simulink model "AWES3_CL_wTether_v4_PM"  (R2022a)
settings: Solver=ode3  StartTime=0  StopTime=simInit.TSIM  FixedStep=simInit.dt  RelTol=1e-3
values from neighbouring files (symbols this model uses):
  complex_tether_flag = 1    [run_sim.m]
  Ft_max = 1870    [run_sim.m]
  q = 0    [barrier_optimization.m]
  r = 0    [barrier_optimization.m]
  random_seed = [ 24335       17059       17670        1747]    [run_sim.m]
  safety_controller = false    [run_sim.m]
  turbulence = true    [run_sim.m]
undefined symbols (not defined in the file or in its folder): aeroModel, alpha_max, alpha_min, alpha_options, base_windspeed, constr, DiscIntNeverNeededParam, dx, ENVMT, F, grid_max, grid_min, HDBK, I_table, Light, MIL, mu_max, mu_min, mu_options, P_AP2, params, SampleTime, simInit, T, u0_sim, winchParameter, x0_sim
libraries: simulink x30, aerolibwind2 x14, dspstat3 x2, pid_lib x1, aerolibwindfilters x1, aerolibcommonsys x1, matrix_library x1
(part 4 of 5)

== system AWES3_CL_wTether_v4_PM/FlightController/Retraction/CalculateAttitudeCmds/FlightpathReferenceModels/SecondOrderReferenceModel_Path2 ==
  y_cmd : Inport
  hedge : Inport  Port=2
  Discrete-Time Integrator : DiscreteIntegrator  InitialCondition=30*pi/180  SampleTime=-1  LimitOutput=on  UpperSaturationLimit=y_max  LowerSaturationLimit=y_min  ICPrevOutput=DiscIntNeverNeededParam  ICPrevScaledInput=DiscIntNeverNeededParam
  Discrete-Time Integrator1 : DiscreteIntegrator  SampleTime=-1  LimitOutput=on  UpperSaturationLimit=yd_max  LowerSaturationLimit=yd_min  ICPrevOutput=DiscIntNeverNeededParam  ICPrevScaledInput=DiscIntNeverNeededParam
  Gain1 : Gain  Gain=omega0^2
  Gain2 : Gain  Gain=2*zeta0*omega0
  Saturation : Saturate  UpperLimit=y_max  LowerLimit=y_min
  Saturation1 : Saturate  UpperLimit=y2d_max  LowerLimit=y2d_min
  Sum : Sum  Inputs=|+-
  Sum1 : Sum  Inputs=|+-
  Sum2 : Sum  Inputs=|+-
  y_ref : Outport  VectorParamsAs1DForOutWhenUnconnected=off
  y_ref_dot : Outport  Port=2  VectorParamsAs1DForOutWhenUnconnected=off
  wires:
  hedge/1 -> Sum2/2
  Sum2/1 -> Discrete-Time Integrator/1
  Saturation/1 -> Sum1/1
  Saturation1/1 -> Discrete-Time Integrator1/1
  Sum1/1 -> Gain1/1
  Gain2/1 -> Sum/2
  Sum/1 -> Saturation1/1
  Discrete-Time Integrator1/1 -> Gain2/1, y_ref_dot/1, Sum2/1
  y_cmd/1 -> Saturation/1
  Gain1/1 -> Sum/1
  Discrete-Time Integrator/1 -> Sum1/2, y_ref/1

== system AWES3_CL_wTether_v4_PM/FlightController/Retraction/CalculateAttitudeCmds/FlightpathReferenceModels/SecondOrderReferenceModel_course ==
  y_cmd : Inport
  hedge : Inport  Port=2
  dynamic_pressure : Inport  Port=3
  Constant : Constant  Value=omega0_max
  Constant1 : Constant  Commented=on  Value=omega0_min
  Constant2 : Constant  Commented=on  Value=dynP_min
  Constant3 : Constant  Commented=on  Value=dynP_max
  Discrete-Time Integrator : DiscreteIntegrator  SampleTime=-1  LimitOutput=on  UpperSaturationLimit=y_max  LowerSaturationLimit=y_min  ICPrevOutput=DiscIntNeverNeededParam  ICPrevScaledInput=DiscIntNeverNeededParam
  Discrete-Time Integrator1 : DiscreteIntegrator  SampleTime=-1  LimitOutput=on  UpperSaturationLimit=yd_max  LowerSaturationLimit=yd_min  ICPrevOutput=DiscIntNeverNeededParam  ICPrevScaledInput=DiscIntNeverNeededParam
  Gain2 : Gain  Gain=2*zeta0
  MATLAB Function : MATLAB Function  Commented=on  TreatAsAtomicUnit=on
  Product : Product  Inputs=3
  Product1 : Product
  Saturation : Saturate  UpperLimit=y_max  LowerLimit=y_min
  Saturation1 : Saturate  UpperLimit=y2d_max  LowerLimit=y2d_min
  Saturation2 : Saturate  Commented=on  UpperLimit=dynP_max  LowerLimit=dynP_min
  Sum : Sum  Inputs=|+-
  Sum2 : Sum  Inputs=|+-
  calcualteCourseErrorAndWrap : MATLAB Function  TreatAsAtomicUnit=on
  wrap2pi2 : MATLAB Function  TreatAsAtomicUnit=on
  y_ref : Outport  VectorParamsAs1DForOutWhenUnconnected=off
  y_ref_dot : Outport  Port=2  VectorParamsAs1DForOutWhenUnconnected=off
  wires:
  Product1/1 -> Gain2/1
  Constant2/1 -> MATLAB Function/5(dynP_min)
  Constant1/1 -> MATLAB Function/2(w0_min)
  dynamic_pressure/1 -> Saturation2/1
  Constant/1 -> Product1/2, Product/3, Product/1
  Constant3/1 -> MATLAB Function/4(dynP_max)
  Saturation2/1 -> MATLAB Function/3(dynP)
  Discrete-Time Integrator/1 -> wrap2pi2/1(u)
  Product/1 -> Sum/1
  y_cmd/1 -> Saturation/1
  Discrete-Time Integrator1/1 -> Sum2/1, y_ref_dot/1, Product1/1  "v:_r"
  Sum/1 -> Saturation1/1
  Gain2/1 -> Sum/2
  calcualteCourseErrorAndWrap/1(e_course) -> Product/2
  Saturation1/1 -> Discrete-Time Integrator1/1  "v_dot_r"
  Saturation/1 -> calcualteCourseErrorAndWrap/1(chi_ref)
  Sum2/1 -> Discrete-Time Integrator/1
  hedge/1 -> Sum2/2
  wrap2pi2/1(y) -> calcualteCourseErrorAndWrap/2(chi), y_ref/1

== system AWES3_CL_wTether_v4_PM/FlightController/Retraction/CalculateAttitudeCmds/FlightpathReferenceModels/SecondOrderReferenceModel_mu_a ==
  y_cmd : Inport
  hedge : Inport  Port=2
  reset : Inport  Port=3
  dynamic_pressure : Inport  Port=4
  Constant : Constant  Value=omega0_max
  Constant1 : Constant  Value=omega0_min
  Constant2 : Constant  Value=dynP_min
  Constant3 : Constant  Value=dynP_max
  Discrete-Time Integrator : DiscreteIntegrator  ExternalReset=rising  SampleTime=-1  LimitOutput=on  UpperSaturationLimit=y_max  LowerSaturationLimit=y_min  ICPrevOutput=DiscIntNeverNeededParam  ICPrevScaledInput=DiscIntNeverNeededParam
  Discrete-Time Integrator1 : DiscreteIntegrator  ExternalReset=rising  SampleTime=-1  LimitOutput=on  UpperSaturationLimit=yd_max  LowerSaturationLimit=yd_min  ICPrevOutput=DiscIntNeverNeededParam  ICPrevScaledInput=DiscIntNeverNeededParam
  Gain2 : Gain  Gain=2*zeta0
  MATLAB Function : MATLAB Function  TreatAsAtomicUnit=on
  Product : Product  Inputs=3
  Product1 : Product
  Saturation : Saturate  UpperLimit=y_max  LowerLimit=y_min
  Saturation1 : Saturate  UpperLimit=y2d_max  LowerLimit=y2d_min
  Saturation2 : Saturate  UpperLimit=dynP_max  LowerLimit=dynP_min
  Sum : Sum  Inputs=|+-
  Sum1 : Sum  Inputs=|+-
  Sum2 : Sum  Inputs=|+-
  y_ref : Outport  VectorParamsAs1DForOutWhenUnconnected=off
  y_ref_dot : Outport  Port=2  VectorParamsAs1DForOutWhenUnconnected=off
  wires:
  Saturation2/1 -> MATLAB Function/3(dynP)
  Product1/1 -> Gain2/1
  MATLAB Function/1(w0_int) -> Product1/2, Product/3, Product/1
  Constant3/1 -> MATLAB Function/4(dynP_max)
  Constant2/1 -> MATLAB Function/5(dynP_min)
  Constant/1 -> MATLAB Function/1(w0_max)
  Constant1/1 -> MATLAB Function/2(w0_min)
  dynamic_pressure/1 -> Saturation2/1
  hedge/1 -> Sum2/2
  Sum2/1 -> Discrete-Time Integrator/1
  Saturation/1 -> Sum1/1
  Saturation1/1 -> Discrete-Time Integrator1/1
  Sum1/1 -> Product/2
  Gain2/1 -> Sum/2
  Sum/1 -> Saturation1/1
  Discrete-Time Integrator1/1 -> y_ref_dot/1, Sum2/1, Product1/1
  y_cmd/1 -> Saturation/1
  Product/1 -> Sum/1
  Discrete-Time Integrator/1 -> y_ref/1, Sum1/2
  reset/1 -> Discrete-Time Integrator/2, Discrete-Time Integrator1/2

== system AWES3_CL_wTether_v4_PM/FlightController/Retraction/CalculateAttitudeCmds/FlightpathReferenceModels/SecondOrderReferenceModel_pathangle ==
  y_cmd : Inport
  hedge : Inport  Port=2
  dynamic_pressure : Inport  Port=3
  Constant : Constant  Value=omega0_max
  Constant1 : Constant  Commented=on  Value=omega0_min
  Constant2 : Constant  Commented=on  Value=dynP_min
  Constant3 : Constant  Commented=on  Value=dynP_max
  Discrete-Time Integrator : DiscreteIntegrator  SampleTime=-1  LimitOutput=on  UpperSaturationLimit=y_max  LowerSaturationLimit=y_min  ICPrevOutput=DiscIntNeverNeededParam  ICPrevScaledInput=DiscIntNeverNeededParam
  Discrete-Time Integrator1 : DiscreteIntegrator  SampleTime=-1  LimitOutput=on  UpperSaturationLimit=yd_max  LowerSaturationLimit=yd_min  ICPrevOutput=DiscIntNeverNeededParam  ICPrevScaledInput=DiscIntNeverNeededParam
  Gain2 : Gain  Gain=2*zeta0
  MATLAB Function : MATLAB Function  Commented=on  TreatAsAtomicUnit=on
  Product : Product  Inputs=3
  Product1 : Product
  Saturation : Saturate  UpperLimit=y_max  LowerLimit=y_min
  Saturation1 : Saturate  UpperLimit=y2d_max  LowerLimit=y2d_min
  Saturation2 : Saturate  Commented=on  UpperLimit=dynP_max  LowerLimit=dynP_min
  Sum : Sum  Inputs=|+-
  Sum1 : Sum  Inputs=|+-
  Sum2 : Sum  Inputs=|+-
  y_ref : Outport  VectorParamsAs1DForOutWhenUnconnected=off
  y_ref_dot : Outport  Port=2  VectorParamsAs1DForOutWhenUnconnected=off
  wires:
  Product1/1 -> Gain2/1
  Constant2/1 -> MATLAB Function/5(dynP_min)
  Constant1/1 -> MATLAB Function/2(w0_min)
  dynamic_pressure/1 -> Saturation2/1
  Constant/1 -> Product/3, Product/1, Product1/2
  Constant3/1 -> MATLAB Function/4(dynP_max)
  Saturation2/1 -> MATLAB Function/3(dynP)
  Product/1 -> Sum/1
  y_cmd/1 -> Saturation/1
  Discrete-Time Integrator1/1 -> Sum2/1, y_ref_dot/1, Product1/1  "v:_r"
  Sum/1 -> Saturation1/1
  Gain2/1 -> Sum/2
  Sum1/1 -> Product/2
  Saturation1/1 -> Discrete-Time Integrator1/1  "v_dot_r"
  Saturation/1 -> Sum1/1
  Sum2/1 -> Discrete-Time Integrator/1
  hedge/1 -> Sum2/2
  Discrete-Time Integrator/1 -> y_ref/1, Sum1/2

== system AWES3_CL_wTether_v4_PM/FlightController/Traction/Ft_set_smoothing/force switch1/Subsystem ==
  Ft : Inport
  dFt : Inport  Port=2
  Constant1 : Constant  Value=Ft_max-40
  Gain : Gain  Gain=-1
  Gain1 : Gain  Gain=-1
  Sum : Sum  Inputs=+-|
  Sum1 : Sum  Inputs=+-|
  mu_1 : Outport
  mu_2 : Outport  Port=2
  mu_3 : Outport  Port=3
  mu_4 : Outport  Port=4
  wires:
  Ft/1 -> Sum/2
  Constant1/1 -> Sum/1
  Sum/1 -> Gain/1, Sum1/1, mu_1/1
  dFt/1 -> Sum1/2
  Sum1/1 -> mu_3/1, Gain1/1
  Gain/1 -> mu_2/1
  Gain1/1 -> mu_4/1

== matlab function AWES3_CL_wTether_v4_PM/Aircraft_Winch_Tether/Subsystem/6DoFKinematics1/AircraftEOM2 ==
  data: M_OB output; v_k_W output; v_w_O input; Va input; alpha input; beta input; mu_a input; F_a_A input; chi_a input; gamma_a input; long input; lat input; h_tau input; P_AP2 parameter; pos_O output; pos_W output; v_k_B output; v_a_dot output; chi_a_dot output; gamma_a_dot output; long_dot output; lat_dot output; h_tau_dot output; chi_k output; gamma_k output; eta_EULER output; v_k_O output; ENVMT parameter; course_tau output; pathangle_tau output; beta_k output; EULER_tau output
function [M_OB, v_k_W, pos_O,pos_W, v_k_B, v_a_dot,chi_a_dot,gamma_a_dot,long_dot,lat_dot,h_tau_dot, chi_k, gamma_k,eta_EULER, v_k_O,  course_tau, pathangle_tau, beta_k, EULER_tau] = ...
    fcn(v_w_O,Va, alpha, beta, mu_a, F_a_A , chi_a, gamma_a, long, lat,h_tau, P_AP2, ENVMT)
beta_k= 0;
alpha_k= 0;
chi_k = 0;
gamma_k  = 0;
M_OB = zeros(3); 
eta_EULER = zeros(3,1); 

%cos_a = cos(alpha); 

M_BA = [cos(alpha), 0, -sin(alpha); 
    0, 1, 0; 
 sin(alpha),0, cos(alpha)];

%M_AB = M_BA.';
M_AB = M_BA';

s_lat = sin(lat); 
s_long = sin(long); 
c_lat = cos(lat); 
c_long = cos(long); 

M_tauW = [-s_lat *c_long, -s_lat *s_long, c_lat;
    -s_long, c_long, 0;
    -c_lat*c_long, -c_lat*s_long, -s_lat ];

xi = ENVMT.windDirection_rad;
M_OW = [cos(xi), sin(xi), 0; 
    sin(xi), -cos(xi), 0; 
    0, 0, -1];
M_WO = M_OW; 

cos_ca = cos(chi_a); 
cos_ga = cos(gamma_a); 
sin_ca = sin(chi_a); 
sin_ga = sin(gamma_a); 

M_AbarO = [cos_ca*cos_ga, sin_ca*cos_ga, -sin_ga; 
    -sin_ca, cos_ca, 0; 
    cos_ca*sin_ga, sin_ca*sin_ga, cos_ga];
M_OAbar = M_AbarO';
M_AbarA = [1,0,0; 
            0, cos(mu_a), -sin(mu_a); 
            0, sin(mu_a), cos(mu_a)];
M_AAbar = M_AbarA';

%%

v_a_O = M_OAbar*[Va;0;0]; 
v_a_B = M_BA*[Va;0;0]; 
%v_w_O = M_OW*v_w_W;
v_w_B = M_BA*M_AAbar*M_AbarO*v_w_O;
v_k_B = v_a_B + v_w_B; 
v_k_O = v_a_O + v_w_O; 
v_k_W = M_WO*v_k_O; 
Vk = norm(v_k_B); 
%beta_k = asin(1/Vk * v_k_B(2) );
beta_k = atan2( v_k_B(2), sqrt( v_k_B(1)^2+v_k_B(3)^2 ) );

%alpha_k = atan2( (v_a_B(3)+v_w_B(3)), (v_a_B(1)+v_w_B(1)) );

chi_k = atan2( v_k_O(2), v_k_O(1) ); 
gamma_k = -asin( 1/Vk*v_k_O(3) ); 


Ftot_Abar = M_AbarA*F_a_A; 

x_dot_Abar = 1/P_AP2.mass*diag([1,1/(Va*cos_ga),-1/Va]) * Ftot_Abar; 
% states are: Va, chi_a, gamma_a
v_a_dot = x_dot_Abar(1); 
chi_a_dot = x_dot_Abar(2);
gamma_a_dot = x_dot_Abar(3); 

v_k_tau =M_tauW*v_k_W;

long_dot = v_k_tau(2)/( abs(h_tau)*cos(lat));
lat_dot = v_k_tau(1)/abs(h_tau);
h_tau_dot = -v_k_tau(3);

pos_W= [cos(long)*cos(lat); sin(long)*cos(lat); sin(lat)]*h_tau;
pos_O = M_OW*pos_W; 
M_OB = M_OAbar * M_AbarA * M_AB;
%%

%%
PHI =  atan2( M_OB(3,2), M_OB(3,3) ); 
THETA = -asin( M_OB(3,1) ); 
PSI = atan2( M_OB(2,1), M_OB(1,1) ); 

eta_EULER = [PHI; THETA; PSI];


%% Tangential plane stuff
M_WO=M_OW';  
M_tauB = M_tauW * M_WO * M_OB; 
%phi_tau = atan2( M_tauB(3,2) , M_tauB(3,3) );
phi_tau = atan( M_tauB(3,2)/M_tauB(3,3) );
theta_tau = -asin( M_tauB(3,1) );
psi_tau = atan2( M_tauB(2,1) , M_tauB(1,1) );
EULER_tau = [phi_tau;theta_tau;psi_tau];

vel_k_tau_mDs = M_tauW * M_OW'*M_OB * v_k_B; 
course_tau = atan2( vel_k_tau_mDs(2), vel_k_tau_mDs(1) ); 
pathangle_tau = [course_tau; -asin( vel_k_tau_mDs(3) / norm( vel_k_tau_mDs ) )];

== matlab function AWES3_CL_wTether_v4_PM/Aircraft_Winch_Tether/ForcesAndMoments1/MATLAB Function ==
  data: F_a_A output; airdata input; P_AP2 parameter; F_a_B output; u_trim input
function [F_a_A, F_a_B] = getAeroForcesAndMoments( airdata,  P_AP2, u_trim )
% Rotational Rates
p =0; 
q = 0; %-0.1202; 
r = 0; 

Va = airdata(1); 
beta = airdata(3); 
alpha = airdata(2);

delta_a = 0*u_trim(1); 
delta_e = u_trim(2); % apparently has quite an impact on the Cx coefficient 
delta_r = 0*u_trim(3); 

%% Force coefficients 
% Cx calculation
Cx_0 = P_AP2.Cx_0_0 + P_AP2.Cx_0_alpha * alpha + P_AP2.Cx_0_alpha2 * alpha^2; 
Cx_q = P_AP2.Cx_q_0 + P_AP2.Cx_q_alpha * alpha + P_AP2.Cx_q_alpha2 * alpha^2; 
Cx_deltaE  = P_AP2.Cx_deltaE_0  + P_AP2.Cx_deltaE_alpha * alpha + P_AP2.Cx_deltaE_alpha2 * alpha^2; 
Cx = Cx_0 + Cx_q*P_AP2.c*q/(2*Va) + Cx_deltaE*delta_e; 

% Cy calculation
Cy_beta = P_AP2.Cy_beta_0 + P_AP2.Cy_beta_alpha * alpha + P_AP2.Cy_beta_alpha2 * alpha^2; 
Cy_p = P_AP2.Cy_p_0  + P_AP2.Cy_p_alpha * alpha + P_AP2.Cy_p_alpha2 * alpha^2;  
Cy_r = P_AP2.Cy_r_0  + P_AP2.Cy_r_alpha * alpha + P_AP2.Cy_r_alpha2 * alpha^2;  
Cy_deltaA =P_AP2.Cy_deltaA_0 + P_AP2.Cy_deltaA_alpha * alpha + P_AP2.Cy_deltaA_alpha2 * alpha^2;  
Cy_deltaR =P_AP2.Cy_deltaR_0 + P_AP2.Cy_deltaR_alpha * alpha + P_AP2.Cy_deltaR_alpha2 * alpha^2;  
Cy = Cy_beta*beta + Cy_p*P_AP2.b*p/(2*Va) + Cy_r*P_AP2.b*r/(2*Va) + Cy_deltaA*delta_a + Cy_deltaR*delta_r;


% Cz calculation
Cz_0 = P_AP2.Cz_0_0 + P_AP2.Cz_0_alpha * alpha + P_AP2.Cz_0_alpha2 * alpha.^2; 
Cz_q = P_AP2.Cz_q_0 + P_AP2.Cz_q_alpha * alpha + P_AP2.Cz_q_alpha2 * alpha^2; 
Cz_deltaE  = P_AP2.Cz_deltaE_0 + P_AP2.Cz_deltaE_alpha * alpha + P_AP2.Cz_deltaE_alpha2 * alpha^2; 
Cz = Cz_0 + Cz_q*P_AP2.c*q/(2*Va) + Cz_deltaE*delta_e; 

F_a_B = 0.5*Va^2*P_AP2.S_ref*1.225* [Cx;Cy; Cz];

M_AB = [cos(alpha)*cos(beta), sin(beta), sin(alpha)*cos(beta); 
    -cos(alpha)*sin(beta), cos(beta), -sin(alpha)*sin(beta); 
    -sin(alpha), 0, cos(alpha)];

F_a_A = M_AB * F_a_B;

% Tether drag calculation. Use only the to the tether perpendicular component 
% of the airspeed
% pos_O = transformFromWtoO(windDirection_rad, pos_W);
% Va_B = M_AB'*[Va;0;0];
% Va_O = DCM*Va_B; 
% t_O = pos_O/norm(pos_O); 
% Va_O_parallel = (Va_O'*t_O)*t_O;
% Va_perp_O = Va_O - Va_O_parallel;
% 
% Dt = 1/8*norm(Va_perp_O)^2*1.225*T.d_tether*T.CD_tether*l_tether;
% F_a_tether_A = [-Dt;0;0];

F_a_A = F_a_A; %+ 0*F_a_tether_A; 
%% Moment coefficients

== matlab function AWES3_CL_wTether_v4_PM/Aircraft_Winch_Tether/ForcesAndMoments1/TetherDragApprox ==
  data: Ftd_A output; airdata input; T parameter; pos_W input; M_OB input; Ftd_A2 output; ENVMT parameter
function [Ftd_A, Ftd_A2]  = fcn(airdata,T, pos_W, M_OB,ENVMT)
Ftd_B = zeros(3,1);
windDirection_rad = ENVMT.windDirection_rad; 

long = atan2( pos_W(2), pos_W(1) ); 
lat = asin( pos_W(3)/norm(pos_W) ); 

Va = airdata(1);
alpha = airdata(2);
beta = airdata(3);

%% For test, delete
% long    = -9.568113232685720e-17;
% lat     = 1.396263401595464;
% h_tau   = 250;
% Va      = 31.346599838167194;
% gamma_a = -0.114668330551869;
% chi_a   = -2.210613291576605;
% 
% alpha   = 0.042840397710006;
% mu_a    = 0.083402612962379;
% 
% M_AbarO = [cos(chi_a) .* cos(gamma_a), sin(chi_a) .* cos(gamma_a), -sin(gamma_a); 
%           -sin(chi_a),                 cos(chi_a),                             0; 
%            cos(chi_a) .* sin(gamma_a), sin(chi_a) .* sin(gamma_a), cos(gamma_a)];
% 
% M_OAbar = M_AbarO';
% M_AbarA = [1,0,0;
%            0, cos(mu_a), -sin(mu_a);
%            0, sin(mu_a), cos(mu_a)];
% 
% M_AB = [cos(alpha) .* cos(beta), sin(beta), sin(alpha) .* cos(beta); 
%     -cos(alpha) .* sin(beta), cos(beta), -sin(alpha) .* sin(beta); 
%     -sin(alpha), 0, cos(alpha)];
% 
% M_OB = M_OAbar * M_AbarA * M_AB;


%%


Phi = atan2( M_OB(3,2), M_OB(3,3) );  
Theta = -asin( M_OB(3,1) ); 

M_AB = [cos(alpha)*cos(beta), sin(beta), sin(alpha)*cos(beta);
    -cos(alpha)*sin(beta), cos(beta), -sin(alpha)*sin(beta);
    -sin(alpha), 0, cos(alpha)];

M_BA = M_AB';
v_a_A = [Va;0;0];
v_a_O = M_OB*M_BA*v_a_A; 

gamma_a = -asin( v_a_O(3)/norm(v_a_O) );

mu_a= asin( max( min( (cos(Theta)*sin(Phi))/(cos(gamma_a)*cos(beta)) + tan(gamma_a) * tan(beta), 1),-1) );

Va_W = transformFromOtoW( windDirection_rad, v_a_O);
M_tauW = [-sin(lat)*cos(long), -sin(lat)*sin(long), cos(lat);
    -sin(long), cos(long), 0;
    -cos(lat)*cos(long), -cos(lat)*sin(long), -sin(lat)];
Va_tau= M_tauW*Va_W;

Fd_tau = -1/8*1.225*T.CD_tether*norm(pos_W)*T.d_tether*sqrt( Va_tau(1)^2 + Va_tau(2)^2 ) * [Va_tau(1); Va_tau(2); 0];

Fd_W = M_tauW'*Fd_tau; %transformFromTautoW( long, lat, Fd_tau);
Fd_O = transformFromWtoO(  windDirection_rad, Fd_W);
Ftd_B2 = M_OB'*Fd_O;% transformFromAbar2B(mu_a, alpha, beta, Fd_Abar );

Ftd_A2 = M_AB*Ftd_B2;
%else
%simplified
Fd_Abar = -1/8*1.225*T.CD_tether*norm(pos_W)*T.d_tether*Va * [Va;0;0];
Ftd_B = transformFromAbar2B(mu_a, alpha, beta, Fd_Abar );

Ftd_A = M_AB*Ftd_B;

end

== stateflow chart AWES3_CL_wTether_v4_PM/HighLevelControlSystem/checkRetractionCondition1 ==
  state calcIncrement1
    during: l_tether_predict =l_tether+l_tether-l0;
  state init2
    entry: init_retraction_flag=1;
  state init
    entry: init_retraction_flag=0;
  state calcIncrement
    during: l_tether_predict =l_tether+l_tether-l0;
  state set0length
    entry: l0 = l_tether;
  calcIncrement1 -> (junction 38) : [path_parameter_s >= (3*pi/2+delta_s_1) && path_parameter_s <=3*pi/2+delta_s_2 ]
  init2 -> init : [fm==6]
  (junction 38) -> init2 [order 1] : [l_tether_predict>=l_tether_max]
  set0length -> calcIncrement1 [order 4] : [path_parameter_s >= (pi/2+delta_s_1) && path_parameter_s <= pi/2+delta_s_2]
  (default) -> init
  set0length -> init [order 2] : [fm==6]
  (junction 38) -> set0length [order 2]
  calcIncrement -> (junction 38) : [path_parameter_s >= (pi/2+delta_s_1) && path_parameter_s <= pi/2+delta_s_2]
  set0length -> init [order 3] : [fm==6]
  init -> set0length : [path_parameter_s >= (pi/2+delta_s_1) && path_parameter_s <= pi/2+delta_s_2 &&fm==5]
  set0length -> calcIncrement [order 1] : [path_parameter_s >= (3*pi/2+delta_s_1) && path_parameter_s <=3*pi/2+delta_s_2]
  data: l_tether input; path_parameter_s input; fm input; l0 local; init_retraction_flag output; l_tether_max input; dl local; l_tether_predict local; delta_s_1 parameter; delta_s_2 parameter

== matlab function AWES3_CL_wTether_v4_PM/Aircraft_Winch_Tether/ForcesAndMoments1/allForcesTorques_exceptAero ==
  data: F_A output; P_AP2 parameter; ENVMT parameter; DCM input; F_t_W input; airdata input; pos_W input; F_t_tot input; Ft_flag input; Ftot output


function [F_A,Ftot]      = forces_moments(P_AP2,ENVMT, DCM,F_t_W, airdata, pos_W, F_t_tot, Ft_flag)

Force = zeros(3,1);
beta = airdata(3);
alpha = airdata(2);
% delta_t = 0;
windDirection_rad = ENVMT.windDirection_rad; 
long = atan2( pos_W(2), pos_W(1) ); 
lat = asin( pos_W(3)/norm(pos_W) ); 

if ~Ft_flag % simple tether
    F_t_W = -[cos(long)*cos(lat);
        sin(long)*cos(lat);
        sin(long)]*F_t_tot;
    F_t_W = -pos_W/norm(pos_W)*F_t_tot;
end

Ftot = norm(F_t_W); 

% Complex tether model force in B
f_kite_G_O = transformFromWtoO(windDirection_rad, F_t_W);

%F_tether_vec_B = f_kite_G_B;
%F_prop_B = [delta_t;0;0];
F_prop_B = zeros(3,1);
% last
F_B = DCM'*([0;0;P_AP2.mass*P_AP2.g]+f_kite_G_O) + F_prop_B;

M_AB = [cos(alpha)*cos(beta), sin(beta), sin(alpha)*cos(beta);
    -cos(alpha)*sin(beta), cos(beta), -sin(alpha)*sin(beta);
    -sin(alpha), 0, cos(alpha)];

F_A = M_AB * F_B;




end

== matlab function AWES3_CL_wTether_v4_PM/Aircraft_Winch_Tether/WindfieldModel/Subsystem1/MATLAB Function1 ==
  data: u input; y output; windDir input
function y = fcn(u, windDir)

%y = transformFromOtoW(windDir,u);

y = zeros(3,1);
M_WO = [cos(windDir), sin(windDir), 0;
        sin(windDir), -cos(windDir), 0;
        0, 0, -1];

y = M_WO*u;

% y(1) = -y(1); 
 %y(3) = -y(3);

== matlab function AWES3_CL_wTether_v4_PM/Aircraft_Winch_Tether/WindfieldModel/Subsystem1/MATLAB Function2 ==
  data: u input; y output; windDir input
function y = fcn(u, windDir)

%y = transformFromOtoW(windDir,u);

y = zeros(3,1);
M_WO = [cos(windDir), sin(windDir), 0;
        sin(windDir), -cos(windDir), 0;
        0, 0, -1];

y = M_WO*u;

% y(1) = -y(1); 
 %y(3) = -y(3);

== matlab function AWES3_CL_wTether_v4_PM/Power/MATLAB Function ==
  data: flag input; m_old input; p_sum input; cnt input; u input; flag output; flightMode input; e_old input; cnt_max_mat input; cycles_cnt input; m_new output; p_sum output; cnt output; e_new output; cnt_max_mat output; cycles_cnt output
% Copyright 2021 Delft University of Technology
%
% Licensed under the Apache License, Version 2.0 (the "License");
% you may not use this file except in compliance with the License.
% You may obtain a copy of the License at
%
%      http://www.apache.org/licenses/LICENSE-2.0
%
% Unless required by applicable law or agreed to in writing, software
% distributed under the License is distributed on an "AS IS" BASIS,
% WITHOUT WARRANTIES OR CONDITIONS OF ANY KIND, either express or implied.
% See the License for the specific language governing permissions and
% limitations under the License.

function [flag, m_new, p_sum, cnt, e_new, cnt_max_mat,cycles_cnt] = fcn(flag, m_old, p_sum, cnt, u, flightMode, e_old,cnt_max_mat,cycles_cnt)

p_sum = p_sum + u;
cnt = cnt + 1;

if flightMode == 5 && flag
    % entering Traction
    cnt_max_mat = cnt; 
    m_new = p_sum/cnt;
    cnt  = 0;
    cycles_cnt = cycles_cnt + 1;
    p_sum = 0;
    flag = 0;
    e_new = abs( m_new - m_old );
elseif flightMode == 6 || flightMode == 7
    % Retraction
    flag = 1;
    m_new = m_old;
    e_new = e_old;
else
    % first Traction
    flag = 0;
    m_new = m_old;
    e_new = e_old;
end

== matlab function AWES3_CL_wTether_v4_PM/FlightController/Traction/Ft_set_smoothing/force switch1/MATLAB Function ==
  data: mu1 input; sigma output; mu2 input; mu3 input; mu4 input; sigma input
function sigma = switching(mu1, mu2, mu3, mu4, sigma)
% sigma = 0: NDI
% sigma = 1: safety
h = 0.10;

if sigma == 0
    if mu1*(1+h) <= min(mu2, mu4) || ...
        mu3*(1+h) <= min(mu2, mu4)
        sigma = 1;
    end
else
    if mu2*(1+h) <= min(mu1, mu3) || ...
        mu4*(1+h) <= min(mu1, mu3)
        sigma = 0;
    end
end

== matlab function AWES3_CL_wTether_v4_PM/FlightController/Traction/Subsystem3/Safety control ==
  data: value output; s input; mu_a output; sigma input; h_tau input; Va input; chi_a input; gamma_a input; tether_diff input; alpha_a output; alpha_options parameter; mu_options parameter; alpha_max parameter; grid_min parameter; grid_max parameter; dx parameter; mu_max parameter; I_table parameter; alpha_min parameter; mu_min parameter
function [value, mu_a, alpha_a] = safetyControl(s, sigma, h_tau, Va, chi_a, gamma_a, tether_diff, alpha_options, mu_options, alpha_max, grid_min, grid_max, dx, mu_max, I_table, alpha_min, mu_min)

    x       = [s, sigma, h_tau, Va, chi_a, gamma_a, tether_diff];
    boundary_min = grid_min' > x;
    boundary_max = grid_max' < x;
    if any(boundary_min) || any(boundary_max)
        value   = false;
        alpha_a = 0;
        mu_a    = 0;
        return
    end
    
    value = true;

    I = eval_u(grid_min, grid_max, dx, I_table, x, 'nearest');
    [I1,I2] = ind2sub([alpha_options, mu_options], I);
    
    alpha_a = alpha_min + (I1-1)/(alpha_options-1) * (alpha_max - alpha_min);
    mu_a    = mu_min    + (I2-1)/(mu_options   -1) * (mu_max    - mu_min);
end    
function v = eval_u(grid_min, grid_max, dx, datas, xs, interp_method)
% Only supporting Single grid, single value function, multiple states
    if nargin < 4
      interp_method = 'linear';
    end
    v = eval_u_single(grid_min, grid_max, dx, datas, xs, interp_method);
end

function v = eval_u_single(grid_min, grid_max, dx, data, x, interp_method)
% v = eval_u_single(g, data, x)
%   Computes the interpolated value of a value function data at state x
%
% Inputs:
%   g       - grid
%   data    - implicit function describing the set
%   x       - points to check; each row is a point
%
% OUTPUT
%   v:  value at points x


%% Dealing with periodicity
% Not implementing now, but should be handled

%% Interpolate
% Input checking
%x = checkInterpInput(g, x);

% Hardcoded for 7 states for now
VS_1 = (grid_min(1) : dx(1) : grid_max(1))';
VS_2 = (grid_min(2) : dx(2) : grid_max(2))';
VS_3 = (grid_min(3) : dx(3) : grid_max(3))';
VS_4 = (grid_min(4) : dx(4) : grid_max(4))';
VS_5 = (grid_min(5) : dx(5) : grid_max(5))';
VS_6 = (grid_min(6) : dx(6) : grid_max(6))';
VS_7 = (grid_min(7) : dx(7) : grid_max(7))';

v = interpn(VS_1, VS_2, VS_3, VS_4, VS_5, VS_6, VS_7, data, ...
            x(1), x(2), x(3), x(4), x(5), x(6), x(7), interp_method);

end

== matlab function AWES3_CL_wTether_v4_PM/Aircraft_Winch_Tether/WindfieldModel/MATLAB Function1 ==
  data: wind_direction_rad input; vec_O output; vec_W input
function vec_O = fcn(wind_direction_rad, vec_W)


M_WO = [cos(wind_direction_rad), sin(wind_direction_rad), 0;
        sin(wind_direction_rad), -cos(wind_direction_rad), 0;
        0, 0, -1];

vec_O = M_WO' * vec_W;

== matlab function AWES3_CL_wTether_v4_PM/Aircraft_Winch_Tether/Subsystem1/MATLAB Function ==
  data: s_dot output; sigma_dot output; F_t_W input; s input; sigma input; long_alt input; lat_alt input; h_tau input; va input; chi_a input; gamma_a input; tether_diff input; alpha input; mu_a input; tether_diff_dot input; v_w_O input; PHI_BOOTH input; long_dot output; lat_dot output; h_tau_dot output; va_dot output; chi_a_dot output; gamma_a_dot output; tether_diff_dot output; T parameter; ENVMT parameter; P_AP2 parameter; base_windspeed parameter; params parameter; F_rest_Abar output
function [s_dot, sigma_dot, long_dot, lat_dot, h_tau_dot, va_dot, chi_a_dot, gamma_a_dot, tether_diff_dot, F_rest_Abar] = ...
    safety_critical_dynamics(F_t_W, s, sigma, long_alt, lat_alt, h_tau, va, chi_a, gamma_a, tether_diff, alpha, mu_a, tether_diff_dot, v_w_O, PHI_BOOTH, T, ENVMT, P_AP2, base_windspeed, params)

% long     = x(1);
% lat      = x(2);
% h_tau    = x(3);
% va       = x(4);
% chi_a    = x(5);
% gamma_a  = x(6);
% tether_diff  = x(7);
% 
% alpha    = u(1);
% mu_a     = u(2);
% l_s_dot  = u(3);
direction = params.direction;
[long, lat, t_tau, t_rot_tau] = getLongLat(s, sigma, h_tau, PHI_BOOTH, params);
% 
% if retraction_flag
%     long = long_alt;
%     lat = lat_alt;
% end
    long = long_alt;
    lat = lat_alt;

beta     = 0;
% Rotational Rates
p = 0; 
q = 0;
r = 0; 

% Hardcoded for now
delta_a = 0; 
delta_e = -0.092174717977942;
delta_r = 0; 

xi      = ENVMT.windDirection_rad;

%% Define rotation matrix
M_AbarA = [1,0,0; 
           0, cos(mu_a), -sin(mu_a); 
           0, sin(mu_a), cos(mu_a)];

M_AB = [cos(alpha) .* cos(beta), sin(beta), sin(alpha) .* cos(beta); 
    -cos(alpha) .* sin(beta), cos(beta), -sin(alpha) .* sin(beta); 
    -sin(alpha), 0, cos(alpha)];

%% Force coefficients 
% Cx calculation
Cx_0 = P_AP2.Cx_0_0 + P_AP2.Cx_0_alpha * alpha + P_AP2.Cx_0_alpha2 * alpha.^2; 
Cx_q = P_AP2.Cx_q_0 + P_AP2.Cx_q_alpha * alpha + P_AP2.Cx_q_alpha2 * alpha.^2; 
Cx_deltaE  = P_AP2.Cx_deltaE_0  + P_AP2.Cx_deltaE_alpha * alpha + P_AP2.Cx_deltaE_alpha2 * alpha.^2; 
Cx = Cx_0 + Cx_q*P_AP2.c*q./(2*va) + Cx_deltaE*delta_e; 

% Cy calculation
Cy_beta = P_AP2.Cy_beta_0 + P_AP2.Cy_beta_alpha * alpha + P_AP2.Cy_beta_alpha2 * alpha.^2; 
Cy_p = P_AP2.Cy_p_0  + P_AP2.Cy_p_alpha * alpha + P_AP2.Cy_p_alpha2 * alpha.^2;  
Cy_r = P_AP2.Cy_r_0  + P_AP2.Cy_r_alpha * alpha + P_AP2.Cy_r_alpha2 * alpha.^2;  
Cy_deltaA = P_AP2.Cy_deltaA_0 + P_AP2.Cy_deltaA_alpha * alpha + P_AP2.Cy_deltaA_alpha2 * alpha.^2;  
Cy_deltaR = P_AP2.Cy_deltaR_0 + P_AP2.Cy_deltaR_alpha * alpha + P_AP2.Cy_deltaR_alpha2 * alpha.^2;  
Cy = Cy_beta*beta + Cy_p*P_AP2.b*p./(2*va) + Cy_r*P_AP2.b*r./(2*va) + Cy_deltaA*delta_a + Cy_deltaR*delta_r;

% Cz calculation
Cz_0 = P_AP2.Cz_0_0 + P_AP2.Cz_0_alpha * alpha + P_AP2.Cz_0_alpha2 * alpha.^2; 
Cz_q = P_AP2.Cz_q_0 + P_AP2.Cz_q_alpha * alpha + P_AP2.Cz_q_alpha2 * alpha.^2; 
Cz_deltaE  = P_AP2.Cz_deltaE_0 + P_AP2.Cz_deltaE_alpha * alpha + P_AP2.Cz_deltaE_alpha2 * alpha.^2; 
Cz = Cz_0 + Cz_q*P_AP2.c*q./(2*va) + Cz_deltaE*delta_e; 

%% Translation Dynamics 
M_tauW = [-sin(lat) .* cos(long), -sin(lat) .* sin(long), cos(lat);
          -sin(long)            , cos(long)             , 0;
          -cos(lat) .* cos(long), -cos(lat) .* sin(long), -sin(lat) ];

M_AbarO = [cos(chi_a) .* cos(gamma_a), sin(chi_a) .* cos(gamma_a), -sin(gamma_a); 
          -sin(chi_a),                 cos(chi_a),                             0; 
           cos(chi_a) .* sin(gamma_a), sin(chi_a) .* sin(gamma_a), cos(gamma_a)];
M_OAbar = M_AbarO';

M_OW = [cos(xi),  sin(xi),  0; 
        sin(xi), -cos(xi),  0; 
        0,              0, -1];
M_WO = M_OW; 

v_a_O = M_OAbar * [va;0;0];
v_k_O = v_a_O + v_w_O; 
v_k_W = M_WO * v_k_O; 

v_k_tau = M_tauW * v_k_W;


s_dot     = 2*pi/945 * t_tau'*v_k_tau./ (direction*norm(t_tau));
sigma_dot = t_rot_tau'*v_k_tau./ (norm(t_tau));

long_dot = (v_k_tau(2))./( abs(h_tau).*cos(lat));
lat_dot = (v_k_tau(1))./abs(h_tau);
h_tau_dot = -(v_k_tau(3));

[pos_W_x,pos_W_y,pos_W_z] = sph2cart(long, lat, h_tau);
pos_W = [pos_W_x; pos_W_y; pos_W_z];
%% Calculate Aerodynamic Forces and Moments
F_a_B = 0.5 * P_AP2.S_ref * 1.225*(va).^2 * [Cx;Cy; Cz];
F_a_A = M_AB * F_a_B;

%% All Forces except Aero
% x_W = [long; lat; h_tau; long_dot; lat_dot; h_tau_dot; tether_diff];
% [f_kite_G_approx , final_seg_diff_dot] = tether_forces(x_W, P_AP2, ENVMT, T, base_windspeed);
%tether_diff_dot = final_seg_diff_dot - l_s_dot;
% F_t_W_approx = -1 * f_kite_G_approx;

%tether_diff_dot = 0;
f_kite_G_O= M_OW * F_t_W;
F_rest_Abar = M_AbarO * ([0;0;P_AP2.mass * ENVMT.g] + f_kite_G_O);

%% Combine all forces
Ftot_Abar = M_AbarA * F_a_A + F_rest_Abar;

va_dot = 1/P_AP2.mass * Ftot_Abar(1);
chi_a_dot  = 1/P_AP2.mass * 1/(va .* cos(gamma_a)) .* Ftot_Abar(2);
gamma_a_dot = 1/P_AP2.mass * -1/(va) .* Ftot_Abar(3);

== matlab function AWES3_CL_wTether_v4_PM/Aircraft_Winch_Tether/Bus Selector/MATLAB Function1 ==
  data: M_OB output; long input; lat input; h_tau input; Va input; chi_a input; gamma_a input; v_k_W output; pos_O output; pos_W output; v_k_B output; Va output; chi_a output; gamma_a output; long output; lat output; h_tau output; chi_k output; gamma_k output; eta_EULER output; v_k_O output; pathangle_tau output; EULER_tau output; alpha_a input; mu_a input; v_w_O input; alpha_a output; ENVMT parameter
function [M_OB, v_k_W, pos_O,pos_W, v_k_B, Va,chi_a,gamma_a,long,lat,h_tau, chi_k, gamma_k,eta_EULER, v_k_O,  pathangle_tau, EULER_tau, alpha_a] = ...
    AricraftBus( long, lat,h_tau, Va, chi_a, gamma_a, alpha_a, mu_a, v_w_O, ENVMT)


M_BA = [cos(alpha_a), 0, -sin(alpha_a); ...
            0, 1, 0; ...
         sin(alpha_a),0, cos(alpha_a)];
M_AB = M_BA';

s_lat = sin(lat); 
s_long = sin(long); 
c_lat = cos(lat); 
c_long = cos(long); 

M_tauW = [-s_lat *c_long, -s_lat *s_long, c_lat;...
    -s_long, c_long, 0;...
    -c_lat*c_long, -c_lat*s_long, -s_lat ];

xi = ENVMT.windDirection_rad;
M_OW = [cos(xi), sin(xi), 0; 
    sin(xi), -cos(xi), 0; 
    0, 0, -1];
M_WO = M_OW; 

cos_ca = cos(chi_a); 
cos_ga = cos(gamma_a); 
sin_ca = sin(chi_a); 
sin_ga = sin(gamma_a); 

M_AbarO = [cos_ca*cos_ga, sin_ca*cos_ga, -sin_ga;  ...
    -sin_ca, cos_ca, 0; ...
    cos_ca*sin_ga, sin_ca*sin_ga, cos_ga];
M_OAbar = M_AbarO';
M_AbarA = [1,0,0; 
            0, cos(mu_a), -sin(mu_a); 
            0, sin(mu_a), cos(mu_a)];
M_AAbar = M_AbarA';

%%

v_a_O = M_OAbar*[Va;0;0]; 
v_a_B = M_BA*[Va;0;0]; 
%v_w_O = M_OW*v_w_W;
v_w_B = M_BA*M_AAbar*M_AbarO*v_w_O;
v_k_B = v_a_B + v_w_B; 
v_k_O = v_a_O + v_w_O; 
v_k_W = M_WO*v_k_O; 
Vk = norm(v_k_B); 

chi_k = atan2( v_k_O(2), v_k_O(1) );
if abs(1/Vk*v_k_O(3)) > 1
    gamma_k = -asin( max(min(1/Vk*v_k_O(3), 1), -1) );
else
    gamma_k = -asin( 1/Vk*v_k_O(3) ); 
end

pos_W= [cos(long)*cos(lat); sin(long)*cos(lat); sin(lat)]*h_tau;
pos_O = M_OW*pos_W; 
M_OB = M_OAbar * M_AbarA * M_AB;

PHI =  atan2( M_OB(3,2), M_OB(3,3) ); 
THETA = -asin( M_OB(3,1) ); 
PSI = atan2( M_OB(2,1), M_OB(1,1) ); 

eta_EULER = [PHI; THETA; PSI];

%% Tangential plane stuff
M_WO=M_OW';  
M_tauB = M_tauW * M_WO * M_OB; 
%phi_tau = atan2( M_tauB(3,2) , M_tauB(3,3) );
phi_tau = atan( M_tauB(3,2)/M_tauB(3,3) );
theta_tau = -asin( M_tauB(3,1) );
psi_tau = atan2( M_tauB(2,1) , M_tauB(1,1) );
EULER_tau = [phi_tau;theta_tau;psi_tau];

vel_k_tau_mDs = M_tauW * M_OW'*M_OB * v_k_B; 
course_tau = atan2( vel_k_tau_mDs(2), vel_k_tau_mDs(1) ); 
pathangle_tau = [course_tau; -asin( vel_k_tau_mDs(3) / norm( vel_k_tau_mDs ) )]; 
end

== matlab function AWES3_CL_wTether_v4_PM/Aircraft_Winch_Tether/WindfieldModel/Subsystem1/MATLAB Function ==
  data: u input; y output; windDir input
function y = fcn(u, windDir)

%y = transformFromOtoW(windDir,u);

y = zeros(3,1);
M_WO = [cos(windDir), sin(windDir), 0;
        sin(windDir), -cos(windDir), 0;
        0, 0, -1];

y = M_WO*u;

% y(1) = -y(1); 
 %y(3) = -y(3);

== matlab function AWES3_CL_wTether_v4_PM/Aircraft_Winch_Tether/ParticleTetherModel/Tethermodel ==
  data: x_dot input; x_dotdot_TetherG2K output; x input; v_ro_set input; l_s input; pos_G_W input; vel_k_G_W input; landedFlag input; l_s_dot output; ground_tether_force output; ENVMT parameter; T parameter; f_kite_G output; vel_W_W_mat input; P_AP2 parameter
function [x_dotdot_TetherG2K,l_s_dot, ground_tether_force,f_kite_G]    = pure_tether_model_function(x_dot, x,...
    v_ro_set,l_s, pos_G_W,vel_k_G_W, landedFlag,ENVMT, T, vel_W_W_mat,P_AP2)
%% Readme
% Equations are adapted from Fechner et al, Dynamic Model of a Pumping Kite
% Power System, Renewable Energy, 2015.
% Implementation: Sebastian Rapp, Wind Energy Institute, Faculty of
% Aerospace Engineering, TU Delft
% Mail: s.rapp@tudelft.nl
% Last change: 19.01.2018
%
% General description:
% This functions calculates the accelerations of the tether particle
% segment based on the acting forces at each particle.
%
% Inputs:
% x_dot: Tether particle velocities (world frame i.e. inertial frame)
% x: Tether particle position (world frame)
% v_w: wind vector (world frame)
% d_tether: tether diameter
% CD_tether: tether drag coefficient
% v_ro_set: reelout speed of the tether
% l_s: tether segment length
% c0: intial spring constant of a tether segment
% d0: initial damping constant of a tether segment
% rho_t: tether mass density (i.e. mass per m)
% g_vec: gravity vector
% rho_air: air density
% x_kite_A,C,D: position bridle attachment points
% xdot_kite_A,C,D: velocities of bridle attachment points
% ls_AKcu,CKcu,DKcu: bridle lengths
% m_kcu: kcu weight
%
% Outputs:
% x_dotdot_TetherG2K: accelertions of the tether particles
% l_s_dot: tether length increases with this speed
% ground_tether_force: tether force as measured at the ground



c0 = T.c0;
d0 = T.d0;
rho_t = P_AP2.rho_tether;% T.rho_t; 
d_tether = P_AP2.d_tether;%  T.d_tether;
CD_tether = P_AP2.Cd_tether;% T.CD_tether;

n_t_p = 5; % amount of particles
l_s_dot = v_ro_set/(n_t_p+1); % Particle speeds

% Adapt stiffness and damping with respect to current segment length
c = c0/max(l_s,60);
d = d0/max(l_s,60);

c = c0/60; 
d = d0/60;

% Mass of tether segments with  respect to current segment length
m = l_s * rho_t;
m_vec = m * ones(n_t_p,1);
%m_vec(n_t_p) = (l_s/2 * rho_t);

p_vec = x;
v_vec = x_dot;
p_norm = zeros(n_t_p,1);

% Vector with distances between particles
p_d = p_vec - [0;0;0; p_vec(1:3*n_t_p-3)];

% Vector with velocity differences
v_d = v_vec - [0;0;0; v_vec(1:3*n_t_p-3)];
%v_d = v_vec - [p_d(1:3)*l_s_dot; v_vec(1:3*n_t_p-3)];

% calculate absolute distances between points
for iter = 1 : n_t_p
    p_norm(iter) = norm( p_d( (iter-1)* 3 + 1 : (iter-1) * 3 + 3 ) );
end

% Gravity vector in W frame
g_vec = [0;0;ENVMT.g];

%%------------------------------- Set up equations of motion-------------------------------
% Initialize matrices
fsd_tot_mat = zeros(3,n_t_p);
x_dotdot = zeros(3,n_t_p);
D_s_mat = zeros(3,n_t_p);

%% Set up equations of motions of ground to kite tether

% Boundary tether force from kite to particle below kite (in the 4p kite model the kcu is connected to the
% points A, C and D

f_kite_G = calcSpringDamperForce( c0,norm( pos_G_W - p_vec(3*(n_t_p) -2 : 3*(n_t_p) ) ), l_s, d0,...
    pos_G_W - p_vec(3*(n_t_p) -2 : 3*(n_t_p) ) ,...
    vel_k_G_W - v_vec( 3*(n_t_p) -2 : 3*(n_t_p)  ) );

 
v_a_p_save = zeros(3, n_t_p);

% Loop through all particles
for idx = 1 : n_t_p
    %v_w_vec = [v_w( idx,: );0;0]+turbulence;
    v_w_vec = vel_W_W_mat(:,idx);
    % Calculate Spring-Damper forces
    fsd_tot_mat(:,idx) = calcSpringDamperForce( c, p_norm(idx), l_s, d, p_d( (idx-1)*3+1:(idx-1)*3+3 ), v_d( (idx-1)*3+1:(idx-1)*3+3) );
    if idx < n_t_p
        fsd_tot_mat(:,idx+1) = calcSpringDamperForce( c, p_norm(idx+1), l_s, d, p_d( idx*3+1:idx*3+3 ), v_d( idx*3+1:idx*3+3) );
    end
    
    % Calculate apparent wind speed of tether particles
    if idx == 1 % Segment that is connected to the ground
        v_a_p = v_w_vec - 0.5*x_dot(1:3) ;
    elseif idx == n_t_p
        v_a_p = v_w_vec - 0.5*( x_dot((idx-2)*3+1:(idx-2)*3+3) + x_dot( (idx-1)*3+1:(idx-1)*3+3) ); % take mean value of adjacent particle vel. for segment velocity
    else
        v_a_p = v_w_vec - 0.5*( x_dot((idx-2)*3+1:(idx-2)*3+3) + x_dot( (idx-1)*3+1:(idx-1)*3+3) ); % take mean value of adjacent particle vel. for segment velocity
    end
    v_a_p_save(1:3, idx) = v_a_p;
    
    % Calculate segment drag
    D_s_mat(:,idx) = 1*calcSegmentDrag(p_d((idx-1)*3+1:(idx-1)*3+3) , v_a_p, ENVMT.rhos, CD_tether, d_tether); % segment drag
    if idx < n_t_p
        % Equations of motion for the groud tether particles Newton x_dotdot = 1/m * (-f + u -mg )
        if idx+1 == n_t_p
            x_dotdot(:,idx) = 1/m_vec(idx) * ( -fsd_tot_mat(:,idx) + 1*fsd_tot_mat(:,idx+1) - m_vec(idx)*g_vec  + D_s_mat(:,idx) );  % Particle dynamics
        else
            if idx == 1
                x_dotdot(:,idx) = 1/m_vec(idx) * ( -fsd_tot_mat(:,1) + fsd_tot_mat(:,2) - m_vec(1)*g_vec  + D_s_mat(:,1) );  % Particle dynamics
            else
                x_dotdot(:,idx) = 1/m_vec(idx) * ( -fsd_tot_mat(:,idx) + 1*fsd_tot_mat(:,idx+1) - m_vec(idx)*g_vec  + D_s_mat(:,idx) );  % Particle dynamics
            end
        end
    else
        % Flexible tether: last particle of the tether is connected to the
        % aircraft CG.
        x_dotdot(:,idx) = 1/m_vec(idx) * ( -1*fsd_tot_mat(:,idx) + f_kite_G - m_vec(idx)*g_vec  + D_s_mat(:,idx) );  % Particle dynamics
    end
    
    ground_tether_force =  fsd_tot_mat(:,1);
    
end

x_dotdot_TetherG2K = reshape(x_dotdot, [3*n_t_p,1]);
if landedFlag
    x_dotdot_TetherG2K = 0 * x_dotdot_TetherG2K;
end


end

== matlab function AWES3_CL_wTether_v4_PM/Aircraft_Winch_Tether/WindfieldModel/MATLAB Function ==
  data: wind_direction_rad input; vec_W output; vec_O input
function vec_W = fcn(wind_direction_rad, vec_O)

vec_W = transformFromOtoW(wind_direction_rad, vec_O);

== matlab function AWES3_CL_wTether_v4_PM/Aircraft_Winch_Tether/WindfieldModel/ShearWind/MATLAB Function ==
  data: v_w_u input; v_w_p_mat output
function v_w_p_mat = fcn(v_w_u)

v_w_p_mat = zeros( 3, length( v_w_u) );
v_w_p_mat(1,:) = v_w_u';

== stateflow chart AWES3_CL_wTether_v4_PM/HighLevelControlSystem/Chart ==
  state AvoidanceFtRup
    entry: mode = 5;
    entry: pathRotFlag = 1;
    during: Ft_set = Ft_set_avoidance;
    during: Pacc = (Pacc+Pin/cnt)*cnt/(cnt+1);
    during: vr_acc = (vr_acc+vr_in);
    during: vr_mean = vr_acc/cnt;
    during: vr_mean_out = vr_mean;
    during: cnt = cnt + 1;
    entry: Ft_set_init = Ft_set_avoidance;
  state StopSim2
    entry:stopSimFlag=1;
  state initTRACTION
    entry: mode = 5;
    entry: cnt = 1;
    entry: Pacc = 0;
    entry: pathRotFlag = 0;
    entry: cycleCounter = 0;
    entry: trac_count = 0;
    during: Ft_set = Ft_set_traction;
    during: Pacc = (Pacc+Pin/cnt)*cnt/(cnt+1);
    during: cnt = cnt + 1;
    entry: Ft_set_init = 1000;
  state TRACTION
    entry: mode = 5;
    entry: pathRotFlag = 1;
    during: Ft_set = Ft_set_traction;
    during: Pacc = (Pacc+Pin/cnt)*cnt/(cnt+1);
    during: vr_acc = (vr_acc+vr_in);
    during: vr_mean = vr_acc/cnt;
    during: vr_mean_out = vr_mean;
    during: cnt = cnt + 1;
  state RETRACTION
    entry: mode = 6;
    during: Ft_set = Ft_set_retraction;
    during: Pacc = (Pacc+Pin/cnt)*cnt/(cnt+1);
    during: cnt = cnt + 1;
    entry: Ft_set_init = Ft_set_retraction;
  state Trans
    entry: trac_count = trac_count + 1;
    entry: mode = 4;
    entry: Ft_set = Ft_set_retraction;
    during: Pacc = (Pacc+Pin/cnt)*cnt/(cnt+1);
    during: cnt = cnt + 1;
  state ApproachTraction
    entry: mode = 7;
    entry: Ft_set = Ft_set_traction;
    entry: Pacc = (Pacc+Pin/cnt)*cnt/(cnt+1);
    entry: cnt = cnt + 1;
    entry: e=abs(Pacc-P_mean_old);
    entry: e_out = e;
    during: Ft_set = Ft_set_traction;
    during: Pacc = (Pacc+Pin/cnt)*cnt/(cnt+1);
    during: cnt = cnt + 1;
    during: e=abs(Pacc-P_mean_old);
    exit: P_mean_old = Pacc;
    exit: cycleCounter = cycleCounter + 1;
    exit: cycleCounter_log = cycleCounter;
  state initTRACTION_4
    entry: mode = 5;
    entry: cnt = 1;
    entry: Pacc = 0;
    entry: pathRotFlag = 0;
    during: Ft_set = Ft_set_traction;
    during: Pacc = (Pacc+Pin/cnt)*cnt/(cnt+1);
    during: cnt = cnt + 1;
  state StopSim1
    entry:stopSimFlag=1;
  TRACTION -> AvoidanceFtRup [order 2] : [avoid_flag==1]
  AvoidanceFtRup -> TRACTION : [avoid_flag==0]
  Trans -> StopSim2 [order 2] : [trac_count>=trac_count_max]
  initTRACTION -> TRACTION : [mod(s,pi)<0.1]
  (default) -> initTRACTION
  Trans -> RETRACTION [order 1] : [Ft<Ft_set_traction*0.8]
  TRACTION -> Trans [order 1] : [initRetractionFlag==1]
  initTRACTION_4 -> TRACTION [order 1] : [mod(s,pi)<0.01]
  RETRACTION -> ApproachTraction : [approachFlag==1]
  ApproachTraction -> initTRACTION_4 : [initTractionFlag==1&&l_t<l_t_min_max]
  initTRACTION_4 -> StopSim1 [order 2] : [cycleCounter>=cycleCounterMax]
  data: initRetractionFlag input; initTractionFlag input; Ft_set output; mode output; Ft_set_traction parameter; Ft_set_retraction parameter; l_t input; l_t_min_max parameter; Ft input; cnt local =1; P_mean_old local =constr.F_t_max*constr.winchParameter.v_max*0.001; Pacc local =0; Pin input; s input; pathRotFlag output; cycleCounterMin parameter; e_conv parameter; stopSimFlag output; cycleCounter local; e local; approachFlag input; cycleCounter_log output; cycleCounterMax parameter; e_out output; vr_in input; Ft_set_traction_low parameter; vr_mean_min parameter; path_rot_complete_flag input; vr_mean local =0; vr_acc local =0; vr_mean_out output; Ft_set_avoidance parameter; avoid_flag input; Ft_set_init output; trac_count local; trac_count_max parameter

== stateflow chart AWES3_CL_wTether_v4_PM/HighLevelControlSystem/checkRetractionCondition ==
  state calcIncrement1
    during: l_tether_predict =l_tether+l_tether-l0;
    during: initiate_trans_retraction_flag = l_tether_predict>=l_tether_max;
  state set0length
    entry: l0 = l_tether;
  state init2
    entry: init_retraction_flag=1;
  state init
    entry: init_retraction_flag=0;
  state calcIncrement
    during: l_tether_predict =l_tether +l_tether-l0;
    during: initiate_trans_retraction_flag = l_tether_predict>=l_tether_max;
  set0length -> calcIncrement1 [order 3] : [path_parameter_s >= (pi/2+delta_s_1) && path_parameter_s <= pi/2+delta_s_2]
  calcIncrement1 -> (junction 38) : [path_parameter_s >= (3*pi/2+delta_s_1) && path_parameter_s <=3*pi/2+delta_s_2 ]
  (junction 38) -> set0length [order 2]
  (junction 38) -> init2 [order 1] : [l_tether_predict>=l_tether_max]
  set0length -> init [order 2] : [fm==6]
  calcIncrement -> (junction 38) : [path_parameter_s >= (pi/2+delta_s_1) && path_parameter_s <= pi/2+delta_s_2]
  (default) -> init
  init2 -> init : [fm==6]
  init -> set0length : [path_parameter_s >= (pi/2+delta_s_1) && path_parameter_s <= pi/2+delta_s_2 &&fm==5]
  set0length -> calcIncrement [order 1] : [path_parameter_s >= (3*pi/2+delta_s_1) && path_parameter_s <=3*pi/2+delta_s_2]
  data: l_tether input; path_parameter_s input; fm input; l0 local; init_retraction_flag output; l_tether_max input; dl local; l_tether_predict local; delta_s_1 parameter; delta_s_2 parameter; initiate_trans_retraction_flag output

== stateflow chart AWES3_CL_wTether_v4_PM/HighLevelControlSystem/Init_Solutions ==
  state SimInit1
    entry: s_init = 3/2*pi;
  state SimInit
    entry: s_init = 2*pi;
  state SimInit2
    entry: s_init = pi/2;
  SimInit1 -> (junction 8) : [mode==6]
  (junction 8) -> SimInit1 [order 1] : [long<=0]
  SimInit -> (junction 8) : [mode==6]
  (default) -> SimInit
  (junction 8) -> SimInit2 [order 2] : [long>0]
  SimInit2 -> (junction 8) : [mode==6]
  data: mode input; long input; s_init output

== matlab function AWES3_CL_wTether_v4_PM/FlightController/Retraction/CalculateAttitudeCmds/FlightPathLoopRetraction/MATLAB Function ==
  data: L_rq output; airdata input; P_AP2 parameter
function L_rq = fcn(airdata, P_AP2)

L_rq =  min( 0.5*P_AP2.rho_air*P_AP2.S_wing*airdata(1)^2 * (P_AP2.CL0+P_AP2.CL_alpha*airdata(2) ),1800); % max. negative lift
